simulink model "bio_matfunc_trapz"  (R2017b)
settings: Solver=VariableStepAuto  StartTime=0.0  StopTime=10.0  RelTol=1e-3
settings Model: Creator=ktrinh  LastModifiedBy=ktrinh

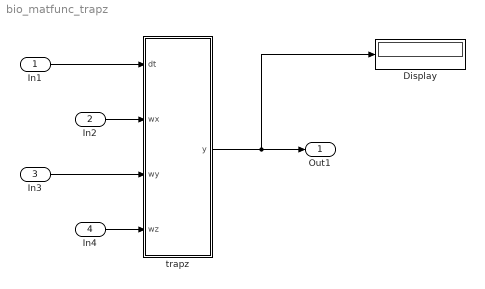
== system bio_matfunc_trapz ==
  In1 : Inport  OutDataTypeStr=double  PortDimensions=1
  In2 : Inport  Port=2  OutDataTypeStr=double  PortDimensions=10
  In3 : Inport  Port=3  OutDataTypeStr=double  PortDimensions=10
  In4 : Inport  Port=4  OutDataTypeStr=double  PortDimensions=10
  Display : Display
  trapz : MATLAB Function  TreatAsAtomicUnit=on
  Out1 : Outport
  wires:
  In1/1 -> trapz/1(dt)
  In2/1 -> trapz/2(wx)
  In3/1 -> trapz/3(wy)
  In4/1 -> trapz/4(wz)
  trapz/1(y) -> Display/1, Out1/1

== matlab function bio_matfunc_trapz/trapz ==
  data: dt input; y output; wx input; wy input; wz input
function y = fcn(dt,wx,wy,wz)
%#codegen

xi = dt*trapz(wx);
yi = dt*trapz(wy);
zi = dt*trapz(wz);

y = [xi;yi;zi];
